simulink model "ex_bus_tutorial_nonvirtual"  (R2017b)
settings: Solver=FixedStepDiscrete  StartTime=0.0  StopTime=10.0  FixedStep=0.200000  RelTol=1e-3
PreLoadFcn:
  | % Bus object: subBus
  | clear elems;
  | elems(1) = Simulink.BusElement;
  | elems(1).Name = 'chirp';
  | elems(1).Dimensions = 2;
  | elems(1).DimensionsMode = 'Fixed';
  | elems(1).DataType = 'double';
  | elems(1).SampleTime = -1;
  | elems(1).Complexity = 'real';
  | elems(1).Min = [];
  | elems(1).Max = [];
  | elems(1).DocUnits = '';
  | elems(1).Description = '';
  | 
  | elems(2) = Simulink.BusElement;
  | elems(2).Name = 'sine';
  | elems(2).Dimensions = 3;
  | elems(2).DimensionsMode = 'Fixed';
  | elems(2).DataType = 'int32';
  | elems(2).SampleTime = -1;
  | elems(2).Complexity = 'real';
  | elems(2).Min = [];
  | elems(2).Max = [];
  | elems(2).DocUnits = '';
  | elems(2).Description = '';
  | 
  | subBus = Simulink.Bus;
  | subBus.HeaderFile = '';
  | subBus.Description = '';
  | subBus.DataScope = 'Auto';
  | subBus.Alignment = -1;
  | subBus.Elements = elems;
  | clear elems;
  | assignin('base','subBus', subBus);
  | 
  | % Bus object: topBus
  | clear elems;
  | elems(1) = Simulink.BusElement;
  | elems(1).Name = 'subSignal';
  | elems(1).Dimensions = 1;
  | elems(1).DimensionsMode = 'Fixed';
  | elems(1).DataType = 'Bus: subBus';
  | elems(1).SampleTime = -1;
  | elems(1).Complexity = 'real';
  | elems(1).Min = [];
  | elems(1).Max = [];
  | elems(1).DocUnits = '';
  | elems(1).Description = '';
  | 
  | elems(2) = Simulink.BusElement;
  | elems(2).Name = 'step';
  | elems(2).Dimensions = 4;
  | elems(2).DimensionsMode = 'Fixed';
  | elems(2).DataType = 'boolean';
  | elems(2).SampleTime = -1;
  | elems(2).Complexity = 'real';
  | elems(2).Min = [];
  | elems(2).Max = [];
  | elems(2).DocUnits = '';
  | elems(2).Description = '';
  | 
  | topBus = Simulink.Bus;
  | topBus.HeaderFile = '';
  | topBus.Description = '';
  | topBus.DataScope = 'Auto';
  | topBus.Alignment = -1;
  | topBus.Elements = elems;
  | clear elems;
  | assignin('base','topBus', topBus);
settings Model: Creator=The MathWorks, Inc.  LastModifiedBy=hbourbou
settings OptimizationCC: LifeSpan=inf
settings DebuggingCC: SFExecutionAtInitializationDiag=none
settings HardwareCC: ProdBitPerSizeT=32  ProdBitPerPtrDiffT=32  ProdWordSize=32  ProdHWDeviceType=Specified
settings CodeAppCC: StateflowObjectComments=on
settings ConfigComp: CovMetricSettings=dswe

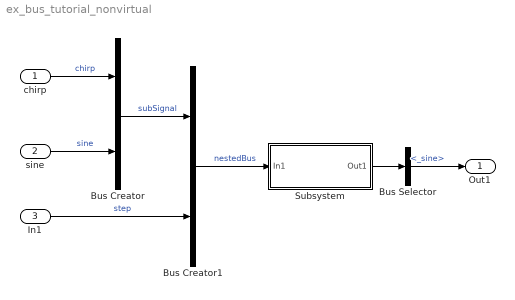
== system ex_bus_tutorial_nonvirtual ==
  chirp : Inport
  sine : Inport  Port=2
  In1 : Inport  Port=3
  Bus Creator1 : BusCreator  Inputs=2  OutDataTypeStr=Bus: topBus  NonVirtualBus=on
      settings: AttributesFormatString=NestedBus
  Bus Selector : BusSelector  OutputSignals=subSignal._sine
  Bus Creator : BusCreator  Inputs=2  OutDataTypeStr=Bus: subBus  NonVirtualBus=on
      settings: AttributesFormatString=SubBus
  Subsystem : Subsystem  TreatAsAtomicUnit=on
  Out1 : Outport
  wires:
  chirp/1 -> Bus Creator/1  "chirp"
  Bus Creator/1 -> Bus Creator1/1  "subSignal"
  Bus Creator1/1 -> Subsystem/1(In1)  "nestedBus"
  sine/1 -> Bus Creator/2  "sine"
  In1/1 -> Bus Creator1/2  "step"
  Subsystem/1(Out1) -> Bus Selector/1
  Bus Selector/1 -> Out1/1  "<_sine>"

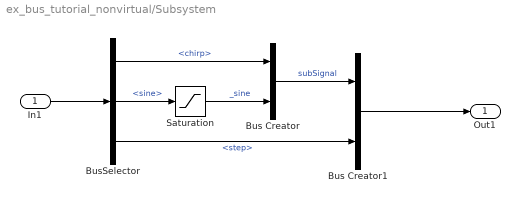
== system ex_bus_tutorial_nonvirtual/Subsystem ==
  In1 : Inport
  Bus Creator : BusCreator  Inputs=2  OutDataTypeStr=Bus: subBus  NonVirtualBus=on
  Bus Creator1 : BusCreator  Inputs=2  OutDataTypeStr=Bus: topBus  NonVirtualBus=on
  BusSelector : BusSelector  OutputSignals=subSignal.chirp,subSignal.sine,step
      settings: AttributesFormatString=BusSelector
  Saturation : Saturate  LowerLimit=-1
  Out1 : Outport
  wires:
  In1/1 -> BusSelector/1
  BusSelector/1 -> Bus Creator/1  "<chirp>"
  BusSelector/2 -> Saturation/1  "<sine>"
  Saturation/1 -> Bus Creator/2  "_sine"
  BusSelector/3 -> Bus Creator1/2  "<step>"
  Bus Creator/1 -> Bus Creator1/1  "subSignal"
  Bus Creator1/1 -> Out1/1
